simulink model "TCMSSystem"  (R2019b)
settings: configuration reference "ConfigSet_TCMSSystem_Reference" (kept outside this file)
model workspace (MAT data in the model file):
  Prm_TCMSSystem : Simulink.Parameter (value not decoded)
  SampleTime = 0.05
symbols that are objects in the model workspace (value not decoded): Prm_TCMSSystem
undefined symbols (not defined in the file): ADDIntervention, AK1Status, AK2Status, AKContactorStatus, AllDoorsClosed, AllLeftDoorsClosed, AllRightDoorsClosed, APS1Fault, APS1Isolated, APS1OutputVoltage, APS1Status, APS2Fault, APS2Isolated, APS2OutputVoltage, APS2Status, APSKAKContactor, ASCOEnd1, ASCOEnd2, ATBMode, ATCBypassMode, ATCStatusNotOK, ATOMode, ATPLowSpeedCutoutStatus, ATPMode, AuxCompressor, BatteryCurrent, BatteryIsolationContactor, BatteryTemperature, BatteryVoltage, BCG1Fault, BCG1Isolated, BCG1IsolationFailed, BCG1OutputCurrent, BCG1Status, BCG2Fault, BCG2Isolated, BCG2OutputCurrent, BCG2Status, BCGOutputVoltage, BECU1AxleLockedWheelSet1, BECU2AxleLockedWheelSet2, BECUFaulty, BECUMajorFault, BECUMinorFault, BECUStatus, BIC1Inside, BIC1Outside, BIC2Inside, BIC2Outside, Bogie, Bogie1WSPStatus, Bogie2WSPStatus, BogieFaulty, BogieIsolationStatus, BogieSupportedMass, BrakeCylinderPressureGauge, BrakeLoopCBTripped, BrakeLoopOpenTL, BrakeTrainLineStatus, BrakingDemand ... (+215)
libraries: TimersLib x257, simulink x137, LatchesLib x42, VectorOperationsLib x15, TestBenchLib x12, MathOperationsLib x2, FiltersLib x1
(part 14 of 16)

== system TCMSSystem/TCMSSystemPerVehicle/EnabledTCMSVehicle/OutputsPacking/TCMSDisplayOutputs/TCMSMessageEvents/ElectricalSystemFaults/Associated TCMS Fault ID37 ==
  State : Inport
  Bus Creator1 : BusCreator  Inputs=2  OutDataTypeStr=Bus: BD_TCMSSystem_Out_Vehicle_Display_Message  NonVirtualBus=on
  Constant : Constant  Value=MessageID
  Data Type Conversion : DataTypeConversion
  Message : Outport  VectorParamsAs1DForOutWhenUnconnected=off
  wires:
  Data Type Conversion/1 -> Bus Creator1/2  "MessageStatus"
  Constant/1 -> Bus Creator1/1  "MessageID"
  State/1 -> Data Type Conversion/1
  Bus Creator1/1 -> Message/1

== system TCMSSystem/TCMSSystemPerVehicle/EnabledTCMSVehicle/OutputsPacking/TCMSDisplayOutputs/TCMSMessageEvents/ElectricalSystemFaults/Associated TCMS Fault ID38 ==
  State : Inport
  Bus Creator1 : BusCreator  Inputs=2  OutDataTypeStr=Bus: BD_TCMSSystem_Out_Vehicle_Display_Message  NonVirtualBus=on
  Constant : Constant  Value=MessageID
  Data Type Conversion : DataTypeConversion
  Message : Outport  VectorParamsAs1DForOutWhenUnconnected=off
  wires:
  Bus Creator1/1 -> Message/1
  State/1 -> Data Type Conversion/1
  Constant/1 -> Bus Creator1/1  "MessageID"
  Data Type Conversion/1 -> Bus Creator1/2  "MessageStatus"

== system TCMSSystem/TCMSSystemPerVehicle/EnabledTCMSVehicle/OutputsPacking/TCMSDisplayOutputs/TCMSMessageEvents/ElectricalSystemFaults/Associated TCMS Fault ID39 ==
  State : Inport
  Bus Creator1 : BusCreator  Inputs=2  OutDataTypeStr=Bus: BD_TCMSSystem_Out_Vehicle_Display_Message  NonVirtualBus=on
  Constant : Constant  Value=MessageID
  Data Type Conversion : DataTypeConversion
  Message : Outport  VectorParamsAs1DForOutWhenUnconnected=off
  wires:
  Bus Creator1/1 -> Message/1
  State/1 -> Data Type Conversion/1
  Constant/1 -> Bus Creator1/1  "MessageID"
  Data Type Conversion/1 -> Bus Creator1/2  "MessageStatus"

== system TCMSSystem/TCMSSystemPerVehicle/EnabledTCMSVehicle/OutputsPacking/TCMSDisplayOutputs/TCMSMessageEvents/ElectricalSystemFaults/Associated TCMS Fault ID4 ==
  State : Inport
  Bus Creator1 : BusCreator  Inputs=2  OutDataTypeStr=Bus: BD_TCMSSystem_Out_Vehicle_Display_Message  NonVirtualBus=on
  Constant : Constant  Value=MessageID
  Data Type Conversion : DataTypeConversion
  Message : Outport  VectorParamsAs1DForOutWhenUnconnected=off
  wires:
  Data Type Conversion/1 -> Bus Creator1/2  "MessageStatus"
  Constant/1 -> Bus Creator1/1  "MessageID"
  State/1 -> Data Type Conversion/1
  Bus Creator1/1 -> Message/1

== system TCMSSystem/TCMSSystemPerVehicle/EnabledTCMSVehicle/OutputsPacking/TCMSDisplayOutputs/TCMSMessageEvents/ElectricalSystemFaults/Associated TCMS Fault ID40 ==
  State : Inport
  Bus Creator1 : BusCreator  Inputs=2  OutDataTypeStr=Bus: BD_TCMSSystem_Out_Vehicle_Display_Message  NonVirtualBus=on
  Constant : Constant  Value=MessageID
  Data Type Conversion : DataTypeConversion
  Message : Outport  VectorParamsAs1DForOutWhenUnconnected=off
  wires:
  Data Type Conversion/1 -> Bus Creator1/2  "MessageStatus"
  Constant/1 -> Bus Creator1/1  "MessageID"
  State/1 -> Data Type Conversion/1
  Bus Creator1/1 -> Message/1

== system TCMSSystem/TCMSSystemPerVehicle/EnabledTCMSVehicle/OutputsPacking/TCMSDisplayOutputs/TCMSMessageEvents/ElectricalSystemFaults/Associated TCMS Fault ID41 ==
  State : Inport
  Bus Creator1 : BusCreator  Inputs=2  OutDataTypeStr=Bus: BD_TCMSSystem_Out_Vehicle_Display_Message  NonVirtualBus=on
  Constant : Constant  Value=MessageID
  Data Type Conversion : DataTypeConversion
  Message : Outport  VectorParamsAs1DForOutWhenUnconnected=off
  wires:
  Bus Creator1/1 -> Message/1
  State/1 -> Data Type Conversion/1
  Constant/1 -> Bus Creator1/1  "MessageID"
  Data Type Conversion/1 -> Bus Creator1/2  "MessageStatus"

== system TCMSSystem/TCMSSystemPerVehicle/EnabledTCMSVehicle/OutputsPacking/TCMSDisplayOutputs/TCMSMessageEvents/ElectricalSystemFaults/Associated TCMS Fault ID42 ==
  State : Inport
  Bus Creator1 : BusCreator  Inputs=2  OutDataTypeStr=Bus: BD_TCMSSystem_Out_Vehicle_Display_Message  NonVirtualBus=on
  Constant : Constant  Value=MessageID
  Data Type Conversion : DataTypeConversion
  Message : Outport  VectorParamsAs1DForOutWhenUnconnected=off
  wires:
  Data Type Conversion/1 -> Bus Creator1/2  "MessageStatus"
  Constant/1 -> Bus Creator1/1  "MessageID"
  State/1 -> Data Type Conversion/1
  Bus Creator1/1 -> Message/1

== system TCMSSystem/TCMSSystemPerVehicle/EnabledTCMSVehicle/OutputsPacking/TCMSDisplayOutputs/TCMSMessageEvents/ElectricalSystemFaults/Associated TCMS Fault ID5 ==
  State : Inport
  Bus Creator1 : BusCreator  Inputs=2  OutDataTypeStr=Bus: BD_TCMSSystem_Out_Vehicle_Display_Message  NonVirtualBus=on
  Constant : Constant  Value=MessageID
  Data Type Conversion : DataTypeConversion
  Message : Outport  VectorParamsAs1DForOutWhenUnconnected=off
  wires:
  Bus Creator1/1 -> Message/1
  State/1 -> Data Type Conversion/1
  Constant/1 -> Bus Creator1/1  "MessageID"
  Data Type Conversion/1 -> Bus Creator1/2  "MessageStatus"

== system TCMSSystem/TCMSSystemPerVehicle/EnabledTCMSVehicle/OutputsPacking/TCMSDisplayOutputs/TCMSMessageEvents/ElectricalSystemFaults/Associated TCMS Fault ID55 ==
  State : Inport
  Bus Creator1 : BusCreator  Inputs=2  OutDataTypeStr=Bus: BD_TCMSSystem_Out_Vehicle_Display_Message  NonVirtualBus=on
  Constant : Constant  Value=MessageID
  Data Type Conversion : DataTypeConversion
  Message : Outport  VectorParamsAs1DForOutWhenUnconnected=off
  wires:
  Bus Creator1/1 -> Message/1
  State/1 -> Data Type Conversion/1
  Constant/1 -> Bus Creator1/1  "MessageID"
  Data Type Conversion/1 -> Bus Creator1/2  "MessageStatus"

== system TCMSSystem/TCMSSystemPerVehicle/EnabledTCMSVehicle/OutputsPacking/TCMSDisplayOutputs/TCMSMessageEvents/ElectricalSystemFaults/Associated TCMS Fault ID56 ==
  State : Inport
  Bus Creator1 : BusCreator  Inputs=2  OutDataTypeStr=Bus: BD_TCMSSystem_Out_Vehicle_Display_Message  NonVirtualBus=on
  Constant : Constant  Value=MessageID
  Data Type Conversion : DataTypeConversion
  Message : Outport  VectorParamsAs1DForOutWhenUnconnected=off
  wires:
  Data Type Conversion/1 -> Bus Creator1/2  "MessageStatus"
  Constant/1 -> Bus Creator1/1  "MessageID"
  State/1 -> Data Type Conversion/1
  Bus Creator1/1 -> Message/1

== system TCMSSystem/TCMSSystemPerVehicle/EnabledTCMSVehicle/OutputsPacking/TCMSDisplayOutputs/TCMSMessageEvents/ElectricalSystemFaults/Associated TCMS Fault ID58 ==
  State : Inport
  Bus Creator1 : BusCreator  Inputs=2  OutDataTypeStr=Bus: BD_TCMSSystem_Out_Vehicle_Display_Message  NonVirtualBus=on
  Constant : Constant  Value=MessageID
  Data Type Conversion : DataTypeConversion
  Message : Outport  VectorParamsAs1DForOutWhenUnconnected=off
  wires:
  Bus Creator1/1 -> Message/1
  State/1 -> Data Type Conversion/1
  Constant/1 -> Bus Creator1/1  "MessageID"
  Data Type Conversion/1 -> Bus Creator1/2  "MessageStatus"

== system TCMSSystem/TCMSSystemPerVehicle/EnabledTCMSVehicle/OutputsPacking/TCMSDisplayOutputs/TCMSMessageEvents/ElectricalSystemFaults/Associated TCMS Fault ID59 ==
  State : Inport
  Bus Creator1 : BusCreator  Inputs=2  OutDataTypeStr=Bus: BD_TCMSSystem_Out_Vehicle_Display_Message  NonVirtualBus=on
  Constant : Constant  Value=MessageID
  Data Type Conversion : DataTypeConversion
  Message : Outport  VectorParamsAs1DForOutWhenUnconnected=off
  wires:
  Data Type Conversion/1 -> Bus Creator1/2  "MessageStatus"
  Constant/1 -> Bus Creator1/1  "MessageID"
  State/1 -> Data Type Conversion/1
  Bus Creator1/1 -> Message/1

== system TCMSSystem/TCMSSystemPerVehicle/EnabledTCMSVehicle/OutputsPacking/TCMSDisplayOutputs/TCMSMessageEvents/ElectricalSystemFaults/Associated TCMS Fault ID6 ==
  State : Inport
  Bus Creator1 : BusCreator  Inputs=2  OutDataTypeStr=Bus: BD_TCMSSystem_Out_Vehicle_Display_Message  NonVirtualBus=on
  Constant : Constant  Value=MessageID
  Data Type Conversion : DataTypeConversion
  Message : Outport  VectorParamsAs1DForOutWhenUnconnected=off
  wires:
  Data Type Conversion/1 -> Bus Creator1/2  "MessageStatus"
  Constant/1 -> Bus Creator1/1  "MessageID"
  State/1 -> Data Type Conversion/1
  Bus Creator1/1 -> Message/1

== system TCMSSystem/TCMSSystemPerVehicle/EnabledTCMSVehicle/OutputsPacking/TCMSDisplayOutputs/TCMSMessageEvents/ElectricalSystemFaults/Associated TCMS Fault ID60 ==
  State : Inport
  Bus Creator1 : BusCreator  Inputs=2  OutDataTypeStr=Bus: BD_TCMSSystem_Out_Vehicle_Display_Message  NonVirtualBus=on
  Constant : Constant  Value=MessageID
  Data Type Conversion : DataTypeConversion
  Message : Outport  VectorParamsAs1DForOutWhenUnconnected=off
  wires:
  Bus Creator1/1 -> Message/1
  State/1 -> Data Type Conversion/1
  Constant/1 -> Bus Creator1/1  "MessageID"
  Data Type Conversion/1 -> Bus Creator1/2  "MessageStatus"

== system TCMSSystem/TCMSSystemPerVehicle/EnabledTCMSVehicle/OutputsPacking/TCMSDisplayOutputs/TCMSMessageEvents/ElectricalSystemFaults/Associated TCMS Fault ID61 ==
  State : Inport
  Bus Creator1 : BusCreator  Inputs=2  OutDataTypeStr=Bus: BD_TCMSSystem_Out_Vehicle_Display_Message  NonVirtualBus=on
  Constant : Constant  Value=MessageID
  Data Type Conversion : DataTypeConversion
  Message : Outport  VectorParamsAs1DForOutWhenUnconnected=off
  wires:
  Data Type Conversion/1 -> Bus Creator1/2  "MessageStatus"
  Constant/1 -> Bus Creator1/1  "MessageID"
  State/1 -> Data Type Conversion/1
  Bus Creator1/1 -> Message/1

== system TCMSSystem/TCMSSystemPerVehicle/EnabledTCMSVehicle/OutputsPacking/TCMSDisplayOutputs/TCMSMessageEvents/ElectricalSystemFaults/Associated TCMS Fault ID62 ==
  State : Inport
  Bus Creator1 : BusCreator  Inputs=2  OutDataTypeStr=Bus: BD_TCMSSystem_Out_Vehicle_Display_Message  NonVirtualBus=on
  Constant : Constant  Value=MessageID
  Data Type Conversion : DataTypeConversion
  Message : Outport  VectorParamsAs1DForOutWhenUnconnected=off
  wires:
  Data Type Conversion/1 -> Bus Creator1/2  "MessageStatus"
  Constant/1 -> Bus Creator1/1  "MessageID"
  State/1 -> Data Type Conversion/1
  Bus Creator1/1 -> Message/1

== system TCMSSystem/TCMSSystemPerVehicle/EnabledTCMSVehicle/OutputsPacking/TCMSDisplayOutputs/TCMSMessageEvents/ElectricalSystemFaults/Associated TCMS Fault ID63 ==
  State : Inport
  Bus Creator1 : BusCreator  Inputs=2  OutDataTypeStr=Bus: BD_TCMSSystem_Out_Vehicle_Display_Message  NonVirtualBus=on
  Constant : Constant  Value=MessageID
  Data Type Conversion : DataTypeConversion
  Message : Outport  VectorParamsAs1DForOutWhenUnconnected=off
  wires:
  Bus Creator1/1 -> Message/1
  State/1 -> Data Type Conversion/1
  Constant/1 -> Bus Creator1/1  "MessageID"
  Data Type Conversion/1 -> Bus Creator1/2  "MessageStatus"

== system TCMSSystem/TCMSSystemPerVehicle/EnabledTCMSVehicle/OutputsPacking/TCMSDisplayOutputs/TCMSMessageEvents/ElectricalSystemFaults/Associated TCMS Fault ID64 ==
  State : Inport
  Bus Creator1 : BusCreator  Inputs=2  OutDataTypeStr=Bus: BD_TCMSSystem_Out_Vehicle_Display_Message  NonVirtualBus=on
  Constant : Constant  Value=MessageID
  Data Type Conversion : DataTypeConversion
  Message : Outport  VectorParamsAs1DForOutWhenUnconnected=off
  wires:
  Data Type Conversion/1 -> Bus Creator1/2  "MessageStatus"
  Constant/1 -> Bus Creator1/1  "MessageID"
  State/1 -> Data Type Conversion/1
  Bus Creator1/1 -> Message/1

== system TCMSSystem/TCMSSystemPerVehicle/EnabledTCMSVehicle/OutputsPacking/TCMSDisplayOutputs/TCMSMessageEvents/ElectricalSystemFaults/Associated TCMS Fault ID65 ==
  State : Inport
  Bus Creator1 : BusCreator  Inputs=2  OutDataTypeStr=Bus: BD_TCMSSystem_Out_Vehicle_Display_Message  NonVirtualBus=on
  Constant : Constant  Value=MessageID
  Data Type Conversion : DataTypeConversion
  Message : Outport  VectorParamsAs1DForOutWhenUnconnected=off
  wires:
  Bus Creator1/1 -> Message/1
  State/1 -> Data Type Conversion/1
  Constant/1 -> Bus Creator1/1  "MessageID"
  Data Type Conversion/1 -> Bus Creator1/2  "MessageStatus"

== system TCMSSystem/TCMSSystemPerVehicle/EnabledTCMSVehicle/OutputsPacking/TCMSDisplayOutputs/TCMSMessageEvents/ElectricalSystemFaults/Associated TCMS Fault ID66 ==
  State : Inport
  Bus Creator1 : BusCreator  Inputs=2  OutDataTypeStr=Bus: BD_TCMSSystem_Out_Vehicle_Display_Message  NonVirtualBus=on
  Constant : Constant  Value=MessageID
  Data Type Conversion : DataTypeConversion
  Message : Outport  VectorParamsAs1DForOutWhenUnconnected=off
  wires:
  Data Type Conversion/1 -> Bus Creator1/2  "MessageStatus"
  Constant/1 -> Bus Creator1/1  "MessageID"
  State/1 -> Data Type Conversion/1
  Bus Creator1/1 -> Message/1

== system TCMSSystem/TCMSSystemPerVehicle/EnabledTCMSVehicle/OutputsPacking/TCMSDisplayOutputs/TCMSMessageEvents/ElectricalSystemFaults/Associated TCMS Fault ID67 ==
  State : Inport
  Bus Creator1 : BusCreator  Inputs=2  OutDataTypeStr=Bus: BD_TCMSSystem_Out_Vehicle_Display_Message  NonVirtualBus=on
  Constant : Constant  Value=MessageID
  Data Type Conversion : DataTypeConversion
  Message : Outport  VectorParamsAs1DForOutWhenUnconnected=off
  wires:
  Bus Creator1/1 -> Message/1
  State/1 -> Data Type Conversion/1
  Constant/1 -> Bus Creator1/1  "MessageID"
  Data Type Conversion/1 -> Bus Creator1/2  "MessageStatus"

== system TCMSSystem/TCMSSystemPerVehicle/EnabledTCMSVehicle/OutputsPacking/TCMSDisplayOutputs/TCMSMessageEvents/ElectricalSystemFaults/Associated TCMS Fault ID68 ==
  State : Inport
  Bus Creator1 : BusCreator  Inputs=2  OutDataTypeStr=Bus: BD_TCMSSystem_Out_Vehicle_Display_Message  NonVirtualBus=on
  Constant : Constant  Value=MessageID
  Data Type Conversion : DataTypeConversion
  Message : Outport  VectorParamsAs1DForOutWhenUnconnected=off
  wires:
  Data Type Conversion/1 -> Bus Creator1/2  "MessageStatus"
  Constant/1 -> Bus Creator1/1  "MessageID"
  State/1 -> Data Type Conversion/1
  Bus Creator1/1 -> Message/1

== system TCMSSystem/TCMSSystemPerVehicle/EnabledTCMSVehicle/OutputsPacking/TCMSDisplayOutputs/TCMSMessageEvents/ElectricalSystemFaults/Associated TCMS Fault ID69 ==
  State : Inport
  Bus Creator1 : BusCreator  Inputs=2  OutDataTypeStr=Bus: BD_TCMSSystem_Out_Vehicle_Display_Message  NonVirtualBus=on
  Constant : Constant  Value=MessageID
  Data Type Conversion : DataTypeConversion
  Message : Outport  VectorParamsAs1DForOutWhenUnconnected=off
  wires:
  Bus Creator1/1 -> Message/1
  State/1 -> Data Type Conversion/1
  Constant/1 -> Bus Creator1/1  "MessageID"
  Data Type Conversion/1 -> Bus Creator1/2  "MessageStatus"

== system TCMSSystem/TCMSSystemPerVehicle/EnabledTCMSVehicle/OutputsPacking/TCMSDisplayOutputs/TCMSMessageEvents/ElectricalSystemFaults/Associated TCMS Fault ID7 ==
  State : Inport
  Bus Creator1 : BusCreator  Inputs=2  OutDataTypeStr=Bus: BD_TCMSSystem_Out_Vehicle_Display_Message  NonVirtualBus=on
  Constant : Constant  Value=MessageID
  Data Type Conversion : DataTypeConversion
  Message : Outport  VectorParamsAs1DForOutWhenUnconnected=off
  wires:
  Bus Creator1/1 -> Message/1
  State/1 -> Data Type Conversion/1
  Constant/1 -> Bus Creator1/1  "MessageID"
  Data Type Conversion/1 -> Bus Creator1/2  "MessageStatus"

== system TCMSSystem/TCMSSystemPerVehicle/EnabledTCMSVehicle/OutputsPacking/TCMSDisplayOutputs/TCMSMessageEvents/ElectricalSystemFaults/Associated TCMS Fault ID70 ==
  State : Inport
  Bus Creator1 : BusCreator  Inputs=2  OutDataTypeStr=Bus: BD_TCMSSystem_Out_Vehicle_Display_Message  NonVirtualBus=on
  Constant : Constant  Value=MessageID
  Data Type Conversion : DataTypeConversion
  Message : Outport  VectorParamsAs1DForOutWhenUnconnected=off
  wires:
  Data Type Conversion/1 -> Bus Creator1/2  "MessageStatus"
  Constant/1 -> Bus Creator1/1  "MessageID"
  State/1 -> Data Type Conversion/1
  Bus Creator1/1 -> Message/1

== system TCMSSystem/TCMSSystemPerVehicle/EnabledTCMSVehicle/OutputsPacking/TCMSDisplayOutputs/TCMSMessageEvents/ElectricalSystemFaults/Associated TCMS Fault ID71 ==
  State : Inport
  Bus Creator1 : BusCreator  Inputs=2  OutDataTypeStr=Bus: BD_TCMSSystem_Out_Vehicle_Display_Message  NonVirtualBus=on
  Constant : Constant  Value=MessageID
  Data Type Conversion : DataTypeConversion
  Message : Outport  VectorParamsAs1DForOutWhenUnconnected=off
  wires:
  Bus Creator1/1 -> Message/1
  State/1 -> Data Type Conversion/1
  Constant/1 -> Bus Creator1/1  "MessageID"
  Data Type Conversion/1 -> Bus Creator1/2  "MessageStatus"

== system TCMSSystem/TCMSSystemPerVehicle/EnabledTCMSVehicle/OutputsPacking/TCMSDisplayOutputs/TCMSMessageEvents/ElectricalSystemFaults/Associated TCMS Fault ID72 ==
  State : Inport
  Bus Creator1 : BusCreator  Inputs=2  OutDataTypeStr=Bus: BD_TCMSSystem_Out_Vehicle_Display_Message  NonVirtualBus=on
  Constant : Constant  Value=MessageID
  Data Type Conversion : DataTypeConversion
  Message : Outport  VectorParamsAs1DForOutWhenUnconnected=off
  wires:
  Data Type Conversion/1 -> Bus Creator1/2  "MessageStatus"
  Constant/1 -> Bus Creator1/1  "MessageID"
  State/1 -> Data Type Conversion/1
  Bus Creator1/1 -> Message/1

== system TCMSSystem/TCMSSystemPerVehicle/EnabledTCMSVehicle/OutputsPacking/TCMSDisplayOutputs/TCMSMessageEvents/ElectricalSystemFaults/Associated TCMS Fault ID73 ==
  State : Inport
  Bus Creator1 : BusCreator  Inputs=2  OutDataTypeStr=Bus: BD_TCMSSystem_Out_Vehicle_Display_Message  NonVirtualBus=on
  Constant : Constant  Value=MessageID
  Data Type Conversion : DataTypeConversion
  Message : Outport  VectorParamsAs1DForOutWhenUnconnected=off
  wires:
  Bus Creator1/1 -> Message/1
  State/1 -> Data Type Conversion/1
  Constant/1 -> Bus Creator1/1  "MessageID"
  Data Type Conversion/1 -> Bus Creator1/2  "MessageStatus"

== system TCMSSystem/TCMSSystemPerVehicle/EnabledTCMSVehicle/OutputsPacking/TCMSDisplayOutputs/TCMSMessageEvents/ElectricalSystemFaults/Associated TCMS Fault ID74 ==
  State : Inport
  Bus Creator1 : BusCreator  Inputs=2  OutDataTypeStr=Bus: BD_TCMSSystem_Out_Vehicle_Display_Message  NonVirtualBus=on
  Constant : Constant  Value=MessageID
  Data Type Conversion : DataTypeConversion
  Message : Outport  VectorParamsAs1DForOutWhenUnconnected=off
  wires:
  Bus Creator1/1 -> Message/1
  State/1 -> Data Type Conversion/1
  Constant/1 -> Bus Creator1/1  "MessageID"
  Data Type Conversion/1 -> Bus Creator1/2  "MessageStatus"

== system TCMSSystem/TCMSSystemPerVehicle/EnabledTCMSVehicle/OutputsPacking/TCMSDisplayOutputs/TCMSMessageEvents/ElectricalSystemFaults/Associated TCMS Fault ID75 ==
  State : Inport
  Bus Creator1 : BusCreator  Inputs=2  OutDataTypeStr=Bus: BD_TCMSSystem_Out_Vehicle_Display_Message  NonVirtualBus=on
  Constant : Constant  Value=MessageID
  Data Type Conversion : DataTypeConversion
  Message : Outport  VectorParamsAs1DForOutWhenUnconnected=off
  wires:
  Data Type Conversion/1 -> Bus Creator1/2  "MessageStatus"
  Constant/1 -> Bus Creator1/1  "MessageID"
  State/1 -> Data Type Conversion/1
  Bus Creator1/1 -> Message/1

== system TCMSSystem/TCMSSystemPerVehicle/EnabledTCMSVehicle/OutputsPacking/TCMSDisplayOutputs/TCMSMessageEvents/ElectricalSystemFaults/Associated TCMS Fault ID76 ==
  State : Inport
  Bus Creator1 : BusCreator  Inputs=2  OutDataTypeStr=Bus: BD_TCMSSystem_Out_Vehicle_Display_Message  NonVirtualBus=on
  Constant : Constant  Value=MessageID
  Data Type Conversion : DataTypeConversion
  Message : Outport  VectorParamsAs1DForOutWhenUnconnected=off
  wires:
  Bus Creator1/1 -> Message/1
  State/1 -> Data Type Conversion/1
  Constant/1 -> Bus Creator1/1  "MessageID"
  Data Type Conversion/1 -> Bus Creator1/2  "MessageStatus"

== system TCMSSystem/TCMSSystemPerVehicle/EnabledTCMSVehicle/OutputsPacking/TCMSDisplayOutputs/TCMSMessageEvents/ElectricalSystemFaults/Associated TCMS Fault ID77 ==
  State : Inport
  Bus Creator1 : BusCreator  Inputs=2  OutDataTypeStr=Bus: BD_TCMSSystem_Out_Vehicle_Display_Message  NonVirtualBus=on
  Constant : Constant  Value=MessageID
  Data Type Conversion : DataTypeConversion
  Message : Outport  VectorParamsAs1DForOutWhenUnconnected=off
  wires:
  Data Type Conversion/1 -> Bus Creator1/2  "MessageStatus"
  Constant/1 -> Bus Creator1/1  "MessageID"
  State/1 -> Data Type Conversion/1
  Bus Creator1/1 -> Message/1

== system TCMSSystem/TCMSSystemPerVehicle/EnabledTCMSVehicle/OutputsPacking/TCMSDisplayOutputs/TCMSMessageEvents/ElectricalSystemFaults/Associated TCMS Fault ID78 ==
  State : Inport
  Bus Creator1 : BusCreator  Inputs=2  OutDataTypeStr=Bus: BD_TCMSSystem_Out_Vehicle_Display_Message  NonVirtualBus=on
  Constant : Constant  Value=MessageID
  Data Type Conversion : DataTypeConversion
  Message : Outport  VectorParamsAs1DForOutWhenUnconnected=off
  wires:
  Bus Creator1/1 -> Message/1
  State/1 -> Data Type Conversion/1
  Constant/1 -> Bus Creator1/1  "MessageID"
  Data Type Conversion/1 -> Bus Creator1/2  "MessageStatus"

== system TCMSSystem/TCMSSystemPerVehicle/EnabledTCMSVehicle/OutputsPacking/TCMSDisplayOutputs/TCMSMessageEvents/ElectricalSystemFaults/Associated TCMS Fault ID79 ==
  State : Inport
  Bus Creator1 : BusCreator  Inputs=2  OutDataTypeStr=Bus: BD_TCMSSystem_Out_Vehicle_Display_Message  NonVirtualBus=on
  Constant : Constant  Value=MessageID
  Data Type Conversion : DataTypeConversion
  Message : Outport  VectorParamsAs1DForOutWhenUnconnected=off
  wires:
  Data Type Conversion/1 -> Bus Creator1/2  "MessageStatus"
  Constant/1 -> Bus Creator1/1  "MessageID"
  State/1 -> Data Type Conversion/1
  Bus Creator1/1 -> Message/1

== system TCMSSystem/TCMSSystemPerVehicle/EnabledTCMSVehicle/OutputsPacking/TCMSDisplayOutputs/TCMSMessageEvents/ElectricalSystemFaults/Associated TCMS Fault ID8 ==
  State : Inport
  Bus Creator1 : BusCreator  Inputs=2  OutDataTypeStr=Bus: BD_TCMSSystem_Out_Vehicle_Display_Message  NonVirtualBus=on
  Constant : Constant  Value=MessageID
  Data Type Conversion : DataTypeConversion
  Message : Outport  VectorParamsAs1DForOutWhenUnconnected=off
  wires:
  Data Type Conversion/1 -> Bus Creator1/2  "MessageStatus"
  Constant/1 -> Bus Creator1/1  "MessageID"
  State/1 -> Data Type Conversion/1
  Bus Creator1/1 -> Message/1

== system TCMSSystem/TCMSSystemPerVehicle/EnabledTCMSVehicle/OutputsPacking/TCMSDisplayOutputs/TCMSMessageEvents/ElectricalSystemFaults/Associated TCMS Fault ID89 ==
  State : Inport
  Bus Creator1 : BusCreator  Inputs=2  OutDataTypeStr=Bus: BD_TCMSSystem_Out_Vehicle_Display_Message  NonVirtualBus=on
  Constant : Constant  Value=MessageID
  Data Type Conversion : DataTypeConversion
  Message : Outport  VectorParamsAs1DForOutWhenUnconnected=off
  wires:
  Bus Creator1/1 -> Message/1
  State/1 -> Data Type Conversion/1
  Constant/1 -> Bus Creator1/1  "MessageID"
  Data Type Conversion/1 -> Bus Creator1/2  "MessageStatus"

== system TCMSSystem/TCMSSystemPerVehicle/EnabledTCMSVehicle/OutputsPacking/TCMSDisplayOutputs/TCMSMessageEvents/ElectricalSystemFaults/Associated TCMS Fault ID9 ==
  State : Inport
  Bus Creator1 : BusCreator  Inputs=2  OutDataTypeStr=Bus: BD_TCMSSystem_Out_Vehicle_Display_Message  NonVirtualBus=on
  Constant : Constant  Value=MessageID
  Data Type Conversion : DataTypeConversion
  Message : Outport  VectorParamsAs1DForOutWhenUnconnected=off
  wires:
  Bus Creator1/1 -> Message/1
  State/1 -> Data Type Conversion/1
  Constant/1 -> Bus Creator1/1  "MessageID"
  Data Type Conversion/1 -> Bus Creator1/2  "MessageStatus"

== system TCMSSystem/TCMSSystemPerVehicle/EnabledTCMSVehicle/OutputsPacking/TCMSDisplayOutputs/TCMSMessageEvents/ElectricalSystemFaults/Associated TCMS Fault ID90 ==
  State : Inport
  Bus Creator1 : BusCreator  Inputs=2  OutDataTypeStr=Bus: BD_TCMSSystem_Out_Vehicle_Display_Message  NonVirtualBus=on
  Constant : Constant  Value=MessageID
  Data Type Conversion : DataTypeConversion
  Message : Outport  VectorParamsAs1DForOutWhenUnconnected=off
  wires:
  Bus Creator1/1 -> Message/1
  State/1 -> Data Type Conversion/1
  Constant/1 -> Bus Creator1/1  "MessageID"
  Data Type Conversion/1 -> Bus Creator1/2  "MessageStatus"

== system TCMSSystem/TCMSSystemPerVehicle/EnabledTCMSVehicle/OutputsPacking/TCMSDisplayOutputs/TCMSMessageEvents/ElectricalSystemFaults/Associated TCMS Fault ID91 ==
  State : Inport
  Bus Creator1 : BusCreator  Inputs=2  OutDataTypeStr=Bus: BD_TCMSSystem_Out_Vehicle_Display_Message  NonVirtualBus=on
  Constant : Constant  Value=MessageID
  Data Type Conversion : DataTypeConversion
  Message : Outport  VectorParamsAs1DForOutWhenUnconnected=off
  wires:
  Data Type Conversion/1 -> Bus Creator1/2  "MessageStatus"
  Constant/1 -> Bus Creator1/1  "MessageID"
  State/1 -> Data Type Conversion/1
  Bus Creator1/1 -> Message/1

== system TCMSSystem/TCMSSystemPerVehicle/EnabledTCMSVehicle/OutputsPacking/TCMSDisplayOutputs/TCMSMessageEvents/ElectricalSystemFaults/Associated TCMS Fault ID92 ==
  State : Inport
  Bus Creator1 : BusCreator  Inputs=2  OutDataTypeStr=Bus: BD_TCMSSystem_Out_Vehicle_Display_Message  NonVirtualBus=on
  Constant : Constant  Value=MessageID
  Data Type Conversion : DataTypeConversion
  Message : Outport  VectorParamsAs1DForOutWhenUnconnected=off
  wires:
  Data Type Conversion/1 -> Bus Creator1/2  "MessageStatus"
  Constant/1 -> Bus Creator1/1  "MessageID"
  State/1 -> Data Type Conversion/1
  Bus Creator1/1 -> Message/1

== system TCMSSystem/TCMSSystemPerVehicle/EnabledTCMSVehicle/OutputsPacking/TCMSDisplayOutputs/TCMSMessageEvents/ElectricalSystemFaults/Associated TCMS Fault ID93 ==
  State : Inport
  Bus Creator1 : BusCreator  Inputs=2  OutDataTypeStr=Bus: BD_TCMSSystem_Out_Vehicle_Display_Message  NonVirtualBus=on
  Constant : Constant  Value=MessageID
  Data Type Conversion : DataTypeConversion
  Message : Outport  VectorParamsAs1DForOutWhenUnconnected=off
  wires:
  Bus Creator1/1 -> Message/1
  State/1 -> Data Type Conversion/1
  Constant/1 -> Bus Creator1/1  "MessageID"
  Data Type Conversion/1 -> Bus Creator1/2  "MessageStatus"

== system TCMSSystem/TCMSSystemPerVehicle/EnabledTCMSVehicle/OutputsPacking/TCMSDisplayOutputs/TCMSMessageEvents/ElectricalSystemFaults/Associated TCMS Fault ID94 ==
  State : Inport
  Bus Creator1 : BusCreator  Inputs=2  OutDataTypeStr=Bus: BD_TCMSSystem_Out_Vehicle_Display_Message  NonVirtualBus=on
  Constant : Constant  Value=MessageID
  Data Type Conversion : DataTypeConversion
  Message : Outport  VectorParamsAs1DForOutWhenUnconnected=off
  wires:
  Data Type Conversion/1 -> Bus Creator1/2  "MessageStatus"
  Constant/1 -> Bus Creator1/1  "MessageID"
  State/1 -> Data Type Conversion/1
  Bus Creator1/1 -> Message/1

== system TCMSSystem/TCMSSystemPerVehicle/EnabledTCMSVehicle/OutputsPacking/TCMSDisplayOutputs/TCMSMessageEvents/ElectricalSystemFaults/Associated TCMS Fault ID95 ==
  State : Inport
  Bus Creator1 : BusCreator  Inputs=2  OutDataTypeStr=Bus: BD_TCMSSystem_Out_Vehicle_Display_Message  NonVirtualBus=on
  Constant : Constant  Value=MessageID
  Data Type Conversion : DataTypeConversion
  Message : Outport  VectorParamsAs1DForOutWhenUnconnected=off
  wires:
  Data Type Conversion/1 -> Bus Creator1/2  "MessageStatus"
  Constant/1 -> Bus Creator1/1  "MessageID"
  State/1 -> Data Type Conversion/1
  Bus Creator1/1 -> Message/1

== system TCMSSystem/TCMSSystemPerVehicle/EnabledTCMSVehicle/OutputsPacking/TCMSDisplayOutputs/TCMSMessageEvents/ElectricalSystemFaults/Associated TCMS Fault ID96 ==
  State : Inport
  Bus Creator1 : BusCreator  Inputs=2  OutDataTypeStr=Bus: BD_TCMSSystem_Out_Vehicle_Display_Message  NonVirtualBus=on
  Constant : Constant  Value=MessageID
  Data Type Conversion : DataTypeConversion
  Message : Outport  VectorParamsAs1DForOutWhenUnconnected=off
  wires:
  Bus Creator1/1 -> Message/1
  State/1 -> Data Type Conversion/1
  Constant/1 -> Bus Creator1/1  "MessageID"
  Data Type Conversion/1 -> Bus Creator1/2  "MessageStatus"

== system TCMSSystem/TCMSSystemPerVehicle/EnabledTCMSVehicle/OutputsPacking/TCMSDisplayOutputs/TCMSMessageEvents/MessageShortList/Associated TCMS Fault ID ==
  State : Inport
  Bus Creator1 : BusCreator  Inputs=2  OutDataTypeStr=Bus: BD_TCMS_Out_Vehicle_Message  NonVirtualBus=on
  Constant : Constant  Value=MessageID
  Data Type Conversion : DataTypeConversion
  Message : Outport  VectorParamsAs1DForOutWhenUnconnected=off
  wires:
  Data Type Conversion/1 -> Bus Creator1/2  "MessageStatus"
  Constant/1 -> Bus Creator1/1  "MessageID"
  State/1 -> Data Type Conversion/1
  Bus Creator1/1 -> Message/1

== system TCMSSystem/TCMSSystemPerVehicle/EnabledTCMSVehicle/OutputsPacking/TCMSDisplayOutputs/TCMSMessageEvents/MessageShortList/For Each Subsystem ==
  Message : Inport  Partition=on  PartitionDimension=1  PartitionWidth=1  PartitionOffset=0
  Bus Selector : BusSelector  OutputSignals=MessageStatus
  For Each : ForEach  DisableCoverage=on
  MessageStatus : Outport  ConcatenationDimension=1
  wires:
  Message/1 -> Bus Selector/1
  Bus Selector/1 -> MessageStatus/1  "<MessageStatus>"

== system TCMSSystem/TCMSSystemPerVehicle/EnabledTCMSVehicle/OutputsPacking/TCMSDisplayOutputs/TCMSMessageEvents/MessageShortList/TCMS Message Index List ==
  note: ensures that events that were
      | previously in the list, don't move
      | around in the order
  note: finds non zero elements pads out to 10 elements
      | 10 is hard coded currently
  Status : Inport
  Delay : Delay  DelayLength=1  InitialCondition=zeros(1,10)
  pad : MATLAB Function  TreatAsAtomicUnit=on
  pad1 : MATLAB Function  TreatAsAtomicUnit=on
  IndexList : Outport  VectorParamsAs1DForOutWhenUnconnected=off
  wires:
  pad/1(y) -> pad1/1(u)
  Delay/1 -> pad1/2(y_prev)
  Status/1 -> pad/1(u)  "status"
  pad1/1(y) -> Delay/1, IndexList/1

== system TCMSSystem/TCMSSystemPerVehicle/EnabledTCMSVehicle/OutputsPacking/TCMSDisplayOutputs/TCMSMessageEvents/MiscellaneousFaults/Associated TCMS Fault ID1 ==
  State : Inport
  Bus Creator1 : BusCreator  Inputs=2  OutDataTypeStr=Bus: BD_TCMSSystem_Out_Vehicle_Display_Message  NonVirtualBus=on
  Constant : Constant  Value=MessageID
  Data Type Conversion : DataTypeConversion
  Message : Outport  VectorParamsAs1DForOutWhenUnconnected=off
  wires:
  Data Type Conversion/1 -> Bus Creator1/2  "MessageStatus"
  Constant/1 -> Bus Creator1/1  "MessageID"
  State/1 -> Data Type Conversion/1
  Bus Creator1/1 -> Message/1

== system TCMSSystem/TCMSSystemPerVehicle/EnabledTCMSVehicle/OutputsPacking/TCMSDisplayOutputs/TCMSMessageEvents/MiscellaneousFaults/Associated TCMS Fault ID102 ==
  State : Inport
  Bus Creator1 : BusCreator  Inputs=2  OutDataTypeStr=Bus: BD_TCMSSystem_Out_Vehicle_Display_Message  NonVirtualBus=on
  Constant : Constant  Value=MessageID
  Data Type Conversion : DataTypeConversion
  Message : Outport  VectorParamsAs1DForOutWhenUnconnected=off
  wires:
  Bus Creator1/1 -> Message/1
  State/1 -> Data Type Conversion/1
  Constant/1 -> Bus Creator1/1  "MessageID"
  Data Type Conversion/1 -> Bus Creator1/2  "MessageStatus"

== system TCMSSystem/TCMSSystemPerVehicle/EnabledTCMSVehicle/OutputsPacking/TCMSDisplayOutputs/TCMSMessageEvents/MiscellaneousFaults/Associated TCMS Fault ID103 ==
  State : Inport
  Bus Creator1 : BusCreator  Inputs=2  OutDataTypeStr=Bus: BD_TCMSSystem_Out_Vehicle_Display_Message  NonVirtualBus=on
  Constant : Constant  Value=MessageID
  Data Type Conversion : DataTypeConversion
  Message : Outport  VectorParamsAs1DForOutWhenUnconnected=off
  wires:
  Data Type Conversion/1 -> Bus Creator1/2  "MessageStatus"
  Constant/1 -> Bus Creator1/1  "MessageID"
  State/1 -> Data Type Conversion/1
  Bus Creator1/1 -> Message/1

== system TCMSSystem/TCMSSystemPerVehicle/EnabledTCMSVehicle/OutputsPacking/TCMSDisplayOutputs/TCMSMessageEvents/MiscellaneousFaults/Associated TCMS Fault ID104 ==
  State : Inport
  Bus Creator1 : BusCreator  Inputs=2  OutDataTypeStr=Bus: BD_TCMSSystem_Out_Vehicle_Display_Message  NonVirtualBus=on
  Constant : Constant  Value=MessageID
  Data Type Conversion : DataTypeConversion
  Message : Outport  VectorParamsAs1DForOutWhenUnconnected=off
  wires:
  Bus Creator1/1 -> Message/1
  State/1 -> Data Type Conversion/1
  Constant/1 -> Bus Creator1/1  "MessageID"
  Data Type Conversion/1 -> Bus Creator1/2  "MessageStatus"

== system TCMSSystem/TCMSSystemPerVehicle/EnabledTCMSVehicle/OutputsPacking/TCMSDisplayOutputs/TCMSMessageEvents/MiscellaneousFaults/Associated TCMS Fault ID105 ==
  State : Inport
  Bus Creator1 : BusCreator  Inputs=2  OutDataTypeStr=Bus: BD_TCMSSystem_Out_Vehicle_Display_Message  NonVirtualBus=on
  Constant : Constant  Value=MessageID
  Data Type Conversion : DataTypeConversion
  Message : Outport  VectorParamsAs1DForOutWhenUnconnected=off
  wires:
  Data Type Conversion/1 -> Bus Creator1/2  "MessageStatus"
  Constant/1 -> Bus Creator1/1  "MessageID"
  State/1 -> Data Type Conversion/1
  Bus Creator1/1 -> Message/1

== system TCMSSystem/TCMSSystemPerVehicle/EnabledTCMSVehicle/OutputsPacking/TCMSDisplayOutputs/TCMSMessageEvents/MiscellaneousFaults/Associated TCMS Fault ID106 ==
  State : Inport
  Bus Creator1 : BusCreator  Inputs=2  OutDataTypeStr=Bus: BD_TCMSSystem_Out_Vehicle_Display_Message  NonVirtualBus=on
  Constant : Constant  Value=MessageID
  Data Type Conversion : DataTypeConversion
  Message : Outport  VectorParamsAs1DForOutWhenUnconnected=off
  wires:
  Bus Creator1/1 -> Message/1
  State/1 -> Data Type Conversion/1
  Constant/1 -> Bus Creator1/1  "MessageID"
  Data Type Conversion/1 -> Bus Creator1/2  "MessageStatus"

== system TCMSSystem/TCMSSystemPerVehicle/EnabledTCMSVehicle/OutputsPacking/TCMSDisplayOutputs/TCMSMessageEvents/MiscellaneousFaults/Associated TCMS Fault ID107 ==
  State : Inport
  Bus Creator1 : BusCreator  Inputs=2  OutDataTypeStr=Bus: BD_TCMSSystem_Out_Vehicle_Display_Message  NonVirtualBus=on
  Constant : Constant  Value=MessageID
  Data Type Conversion : DataTypeConversion
  Message : Outport  VectorParamsAs1DForOutWhenUnconnected=off
  wires:
  Data Type Conversion/1 -> Bus Creator1/2  "MessageStatus"
  Constant/1 -> Bus Creator1/1  "MessageID"
  State/1 -> Data Type Conversion/1
  Bus Creator1/1 -> Message/1

== system TCMSSystem/TCMSSystemPerVehicle/EnabledTCMSVehicle/OutputsPacking/TCMSDisplayOutputs/TCMSMessageEvents/MiscellaneousFaults/Associated TCMS Fault ID108 ==
  State : Inport
  Bus Creator1 : BusCreator  Inputs=2  OutDataTypeStr=Bus: BD_TCMSSystem_Out_Vehicle_Display_Message  NonVirtualBus=on
  Constant : Constant  Value=MessageID
  Data Type Conversion : DataTypeConversion
  Message : Outport  VectorParamsAs1DForOutWhenUnconnected=off
  wires:
  Bus Creator1/1 -> Message/1
  State/1 -> Data Type Conversion/1
  Constant/1 -> Bus Creator1/1  "MessageID"
  Data Type Conversion/1 -> Bus Creator1/2  "MessageStatus"

== system TCMSSystem/TCMSSystemPerVehicle/EnabledTCMSVehicle/OutputsPacking/TCMSDisplayOutputs/TCMSMessageEvents/New46EventsMessage/Associated TCMS Fault ID1 ==
  State : Inport
  Bus Creator1 : BusCreator  Inputs=2  OutDataTypeStr=Bus: BD_TCMSSystem_Out_Vehicle_Display_Message  NonVirtualBus=on
  Constant : Constant  Value=MessageID
  Data Type Conversion : DataTypeConversion
  Message : Outport  VectorParamsAs1DForOutWhenUnconnected=off
  wires:
  Bus Creator1/1 -> Message/1
  State/1 -> Data Type Conversion/1
  Constant/1 -> Bus Creator1/1  "MessageID"
  Data Type Conversion/1 -> Bus Creator1/2  "MessageStatus"

== system TCMSSystem/TCMSSystemPerVehicle/EnabledTCMSVehicle/OutputsPacking/TCMSDisplayOutputs/TCMSMessageEvents/New46EventsMessage/Associated TCMS Fault ID11 ==
  State : Inport
  Bus Creator1 : BusCreator  Inputs=2  OutDataTypeStr=Bus: BD_TCMSSystem_Out_Vehicle_Display_Message  NonVirtualBus=on
  Constant : Constant  Value=MessageID
  Data Type Conversion : DataTypeConversion
  Message : Outport  VectorParamsAs1DForOutWhenUnconnected=off
  wires:
  Bus Creator1/1 -> Message/1
  State/1 -> Data Type Conversion/1
  Constant/1 -> Bus Creator1/1  "MessageID"
  Data Type Conversion/1 -> Bus Creator1/2  "MessageStatus"

== system TCMSSystem/TCMSSystemPerVehicle/EnabledTCMSVehicle/OutputsPacking/TCMSDisplayOutputs/TCMSMessageEvents/New46EventsMessage/Associated TCMS Fault ID12 ==
  State : Inport
  Bus Creator1 : BusCreator  Inputs=2  OutDataTypeStr=Bus: BD_TCMSSystem_Out_Vehicle_Display_Message  NonVirtualBus=on
  Constant : Constant  Value=MessageID
  Data Type Conversion : DataTypeConversion
  Message : Outport  VectorParamsAs1DForOutWhenUnconnected=off
  wires:
  Bus Creator1/1 -> Message/1
  State/1 -> Data Type Conversion/1
  Constant/1 -> Bus Creator1/1  "MessageID"
  Data Type Conversion/1 -> Bus Creator1/2  "MessageStatus"

== system TCMSSystem/TCMSSystemPerVehicle/EnabledTCMSVehicle/OutputsPacking/TCMSDisplayOutputs/TCMSMessageEvents/New46EventsMessage/Associated TCMS Fault ID16 ==
  State : Inport
  Bus Creator1 : BusCreator  Inputs=2  OutDataTypeStr=Bus: BD_TCMSSystem_Out_Vehicle_Display_Message  NonVirtualBus=on
  Constant : Constant  Value=MessageID
  Data Type Conversion : DataTypeConversion
  Message : Outport  VectorParamsAs1DForOutWhenUnconnected=off
  wires:
  Bus Creator1/1 -> Message/1
  State/1 -> Data Type Conversion/1
  Constant/1 -> Bus Creator1/1  "MessageID"
  Data Type Conversion/1 -> Bus Creator1/2  "MessageStatus"

== system TCMSSystem/TCMSSystemPerVehicle/EnabledTCMSVehicle/OutputsPacking/TCMSDisplayOutputs/TCMSMessageEvents/New46EventsMessage/Associated TCMS Fault ID17 ==
  State : Inport
  Bus Creator1 : BusCreator  Inputs=2  OutDataTypeStr=Bus: BD_TCMSSystem_Out_Vehicle_Display_Message  NonVirtualBus=on
  Constant : Constant  Value=MessageID
  Data Type Conversion : DataTypeConversion
  Message : Outport  VectorParamsAs1DForOutWhenUnconnected=off
  wires:
  Data Type Conversion/1 -> Bus Creator1/2  "MessageStatus"
  Constant/1 -> Bus Creator1/1  "MessageID"
  State/1 -> Data Type Conversion/1
  Bus Creator1/1 -> Message/1

== system TCMSSystem/TCMSSystemPerVehicle/EnabledTCMSVehicle/OutputsPacking/TCMSDisplayOutputs/TCMSMessageEvents/New46EventsMessage/Associated TCMS Fault ID18 ==
  State : Inport
  Bus Creator1 : BusCreator  Inputs=2  OutDataTypeStr=Bus: BD_TCMSSystem_Out_Vehicle_Display_Message  NonVirtualBus=on
  Constant : Constant  Value=MessageID
  Data Type Conversion : DataTypeConversion
  Message : Outport  VectorParamsAs1DForOutWhenUnconnected=off
  wires:
  Data Type Conversion/1 -> Bus Creator1/2  "MessageStatus"
  Constant/1 -> Bus Creator1/1  "MessageID"
  State/1 -> Data Type Conversion/1
  Bus Creator1/1 -> Message/1

== system TCMSSystem/TCMSSystemPerVehicle/EnabledTCMSVehicle/OutputsPacking/TCMSDisplayOutputs/TCMSMessageEvents/New46EventsMessage/Associated TCMS Fault ID19 ==
  State : Inport
  Bus Creator1 : BusCreator  Inputs=2  OutDataTypeStr=Bus: BD_TCMSSystem_Out_Vehicle_Display_Message  NonVirtualBus=on
  Constant : Constant  Value=MessageID
  Data Type Conversion : DataTypeConversion
  Message : Outport  VectorParamsAs1DForOutWhenUnconnected=off
  wires:
  Bus Creator1/1 -> Message/1
  State/1 -> Data Type Conversion/1
  Constant/1 -> Bus Creator1/1  "MessageID"
  Data Type Conversion/1 -> Bus Creator1/2  "MessageStatus"

== system TCMSSystem/TCMSSystemPerVehicle/EnabledTCMSVehicle/OutputsPacking/TCMSDisplayOutputs/TCMSMessageEvents/New46EventsMessage/Associated TCMS Fault ID2 ==
  State : Inport
  Bus Creator1 : BusCreator  Inputs=2  OutDataTypeStr=Bus: BD_TCMSSystem_Out_Vehicle_Display_Message  NonVirtualBus=on
  Constant : Constant  Value=MessageID
  Data Type Conversion : DataTypeConversion
  Message : Outport  VectorParamsAs1DForOutWhenUnconnected=off
  wires:
  Data Type Conversion/1 -> Bus Creator1/2  "MessageStatus"
  Constant/1 -> Bus Creator1/1  "MessageID"
  State/1 -> Data Type Conversion/1
  Bus Creator1/1 -> Message/1

== system TCMSSystem/TCMSSystemPerVehicle/EnabledTCMSVehicle/OutputsPacking/TCMSDisplayOutputs/TCMSMessageEvents/New46EventsMessage/Associated TCMS Fault ID20 ==
  State : Inport
  Bus Creator1 : BusCreator  Inputs=2  OutDataTypeStr=Bus: BD_TCMSSystem_Out_Vehicle_Display_Message  NonVirtualBus=on
  Constant : Constant  Value=MessageID
  Data Type Conversion : DataTypeConversion
  Message : Outport  VectorParamsAs1DForOutWhenUnconnected=off
  wires:
  Data Type Conversion/1 -> Bus Creator1/2  "MessageStatus"
  Constant/1 -> Bus Creator1/1  "MessageID"
  State/1 -> Data Type Conversion/1
  Bus Creator1/1 -> Message/1

== system TCMSSystem/TCMSSystemPerVehicle/EnabledTCMSVehicle/OutputsPacking/TCMSDisplayOutputs/TCMSMessageEvents/New46EventsMessage/Associated TCMS Fault ID21 ==
  State : Inport
  Bus Creator1 : BusCreator  Inputs=2  OutDataTypeStr=Bus: BD_TCMSSystem_Out_Vehicle_Display_Message  NonVirtualBus=on
  Constant : Constant  Value=MessageID
  Data Type Conversion : DataTypeConversion
  Message : Outport  VectorParamsAs1DForOutWhenUnconnected=off
  wires:
  Bus Creator1/1 -> Message/1
  State/1 -> Data Type Conversion/1
  Constant/1 -> Bus Creator1/1  "MessageID"
  Data Type Conversion/1 -> Bus Creator1/2  "MessageStatus"

== system TCMSSystem/TCMSSystemPerVehicle/EnabledTCMSVehicle/OutputsPacking/TCMSDisplayOutputs/TCMSMessageEvents/New46EventsMessage/Associated TCMS Fault ID23 ==
  State : Inport
  Bus Creator1 : BusCreator  Inputs=2  OutDataTypeStr=Bus: BD_TCMSSystem_Out_Vehicle_Display_Message  NonVirtualBus=on
  Constant : Constant  Value=MessageID
  Data Type Conversion : DataTypeConversion
  Message : Outport  VectorParamsAs1DForOutWhenUnconnected=off
  wires:
  Bus Creator1/1 -> Message/1
  State/1 -> Data Type Conversion/1
  Constant/1 -> Bus Creator1/1  "MessageID"
  Data Type Conversion/1 -> Bus Creator1/2  "MessageStatus"

== system TCMSSystem/TCMSSystemPerVehicle/EnabledTCMSVehicle/OutputsPacking/TCMSDisplayOutputs/TCMSMessageEvents/New46EventsMessage/Associated TCMS Fault ID24 ==
  State : Inport
  Bus Creator1 : BusCreator  Inputs=2  OutDataTypeStr=Bus: BD_TCMSSystem_Out_Vehicle_Display_Message  NonVirtualBus=on
  Constant : Constant  Value=MessageID
  Data Type Conversion : DataTypeConversion
  Message : Outport  VectorParamsAs1DForOutWhenUnconnected=off
  wires:
  Data Type Conversion/1 -> Bus Creator1/2  "MessageStatus"
  Constant/1 -> Bus Creator1/1  "MessageID"
  State/1 -> Data Type Conversion/1
  Bus Creator1/1 -> Message/1

== system TCMSSystem/TCMSSystemPerVehicle/EnabledTCMSVehicle/OutputsPacking/TCMSDisplayOutputs/TCMSMessageEvents/New46EventsMessage/Associated TCMS Fault ID25 ==
  State : Inport
  Bus Creator1 : BusCreator  Inputs=2  OutDataTypeStr=Bus: BD_TCMSSystem_Out_Vehicle_Display_Message  NonVirtualBus=on
  Constant : Constant  Value=MessageID
  Data Type Conversion : DataTypeConversion
  Message : Outport  VectorParamsAs1DForOutWhenUnconnected=off
  wires:
  Bus Creator1/1 -> Message/1
  State/1 -> Data Type Conversion/1
  Constant/1 -> Bus Creator1/1  "MessageID"
  Data Type Conversion/1 -> Bus Creator1/2  "MessageStatus"

== system TCMSSystem/TCMSSystemPerVehicle/EnabledTCMSVehicle/OutputsPacking/TCMSDisplayOutputs/TCMSMessageEvents/New46EventsMessage/Associated TCMS Fault ID26 ==
  State : Inport
  Bus Creator1 : BusCreator  Inputs=2  OutDataTypeStr=Bus: BD_TCMSSystem_Out_Vehicle_Display_Message  NonVirtualBus=on
  Constant : Constant  Value=MessageID
  Data Type Conversion : DataTypeConversion
  Message : Outport  VectorParamsAs1DForOutWhenUnconnected=off
  wires:
  Data Type Conversion/1 -> Bus Creator1/2  "MessageStatus"
  Constant/1 -> Bus Creator1/1  "MessageID"
  State/1 -> Data Type Conversion/1
  Bus Creator1/1 -> Message/1

== system TCMSSystem/TCMSSystemPerVehicle/EnabledTCMSVehicle/OutputsPacking/TCMSDisplayOutputs/TCMSMessageEvents/New46EventsMessage/Associated TCMS Fault ID27 ==
  State : Inport
  Bus Creator1 : BusCreator  Inputs=2  OutDataTypeStr=Bus: BD_TCMSSystem_Out_Vehicle_Display_Message  NonVirtualBus=on
  Constant : Constant  Value=MessageID
  Data Type Conversion : DataTypeConversion
  Message : Outport  VectorParamsAs1DForOutWhenUnconnected=off
  wires:
  Data Type Conversion/1 -> Bus Creator1/2  "MessageStatus"
  Constant/1 -> Bus Creator1/1  "MessageID"
  State/1 -> Data Type Conversion/1
  Bus Creator1/1 -> Message/1

== system TCMSSystem/TCMSSystemPerVehicle/EnabledTCMSVehicle/OutputsPacking/TCMSDisplayOutputs/TCMSMessageEvents/New46EventsMessage/Associated TCMS Fault ID28 ==
  State : Inport
  Bus Creator1 : BusCreator  Inputs=2  OutDataTypeStr=Bus: BD_TCMSSystem_Out_Vehicle_Display_Message  NonVirtualBus=on
  Constant : Constant  Value=MessageID
  Data Type Conversion : DataTypeConversion
  Message : Outport  VectorParamsAs1DForOutWhenUnconnected=off
  wires:
  Data Type Conversion/1 -> Bus Creator1/2  "MessageStatus"
  Constant/1 -> Bus Creator1/1  "MessageID"
  State/1 -> Data Type Conversion/1
  Bus Creator1/1 -> Message/1

== system TCMSSystem/TCMSSystemPerVehicle/EnabledTCMSVehicle/OutputsPacking/TCMSDisplayOutputs/TCMSMessageEvents/New46EventsMessage/Associated TCMS Fault ID29 ==
  State : Inport
  Bus Creator1 : BusCreator  Inputs=2  OutDataTypeStr=Bus: BD_TCMSSystem_Out_Vehicle_Display_Message  NonVirtualBus=on
  Constant : Constant  Value=MessageID
  Data Type Conversion : DataTypeConversion
  Message : Outport  VectorParamsAs1DForOutWhenUnconnected=off
  wires:
  Bus Creator1/1 -> Message/1
  State/1 -> Data Type Conversion/1
  Constant/1 -> Bus Creator1/1  "MessageID"
  Data Type Conversion/1 -> Bus Creator1/2  "MessageStatus"

== system TCMSSystem/TCMSSystemPerVehicle/EnabledTCMSVehicle/OutputsPacking/TCMSDisplayOutputs/TCMSMessageEvents/New46EventsMessage/Associated TCMS Fault ID3 ==
  State : Inport
  Bus Creator1 : BusCreator  Inputs=2  OutDataTypeStr=Bus: BD_TCMSSystem_Out_Vehicle_Display_Message  NonVirtualBus=on
  Constant : Constant  Value=MessageID
  Data Type Conversion : DataTypeConversion
  Message : Outport  VectorParamsAs1DForOutWhenUnconnected=off
  wires:
  Bus Creator1/1 -> Message/1
  State/1 -> Data Type Conversion/1
  Constant/1 -> Bus Creator1/1  "MessageID"
  Data Type Conversion/1 -> Bus Creator1/2  "MessageStatus"

== system TCMSSystem/TCMSSystemPerVehicle/EnabledTCMSVehicle/OutputsPacking/TCMSDisplayOutputs/TCMSMessageEvents/New46EventsMessage/Associated TCMS Fault ID30 ==
  State : Inport
  Bus Creator1 : BusCreator  Inputs=2  OutDataTypeStr=Bus: BD_TCMSSystem_Out_Vehicle_Display_Message  NonVirtualBus=on
  Constant : Constant  Value=MessageID
  Data Type Conversion : DataTypeConversion
  Message : Outport  VectorParamsAs1DForOutWhenUnconnected=off
  wires:
  Data Type Conversion/1 -> Bus Creator1/2  "MessageStatus"
  Constant/1 -> Bus Creator1/1  "MessageID"
  State/1 -> Data Type Conversion/1
  Bus Creator1/1 -> Message/1

== system TCMSSystem/TCMSSystemPerVehicle/EnabledTCMSVehicle/OutputsPacking/TCMSDisplayOutputs/TCMSMessageEvents/New46EventsMessage/Associated TCMS Fault ID31 ==
  State : Inport
  Bus Creator1 : BusCreator  Inputs=2  OutDataTypeStr=Bus: BD_TCMSSystem_Out_Vehicle_Display_Message  NonVirtualBus=on
  Constant : Constant  Value=MessageID
  Data Type Conversion : DataTypeConversion
  Message : Outport  VectorParamsAs1DForOutWhenUnconnected=off
  wires:
  Bus Creator1/1 -> Message/1
  State/1 -> Data Type Conversion/1
  Constant/1 -> Bus Creator1/1  "MessageID"
  Data Type Conversion/1 -> Bus Creator1/2  "MessageStatus"

== system TCMSSystem/TCMSSystemPerVehicle/EnabledTCMSVehicle/OutputsPacking/TCMSDisplayOutputs/TCMSMessageEvents/New46EventsMessage/Associated TCMS Fault ID34 ==
  State : Inport
  Bus Creator1 : BusCreator  Inputs=2  OutDataTypeStr=Bus: BD_TCMSSystem_Out_Vehicle_Display_Message  NonVirtualBus=on
  Constant : Constant  Value=MessageID
  Data Type Conversion : DataTypeConversion
  Message : Outport  VectorParamsAs1DForOutWhenUnconnected=off
  wires:
  Bus Creator1/1 -> Message/1
  State/1 -> Data Type Conversion/1
  Constant/1 -> Bus Creator1/1  "MessageID"
  Data Type Conversion/1 -> Bus Creator1/2  "MessageStatus"

== system TCMSSystem/TCMSSystemPerVehicle/EnabledTCMSVehicle/OutputsPacking/TCMSDisplayOutputs/TCMSMessageEvents/New46EventsMessage/Associated TCMS Fault ID37 ==
  State : Inport
  Bus Creator1 : BusCreator  Inputs=2  OutDataTypeStr=Bus: BD_TCMSSystem_Out_Vehicle_Display_Message  NonVirtualBus=on
  Constant : Constant  Value=MessageID
  Data Type Conversion : DataTypeConversion
  Message : Outport  VectorParamsAs1DForOutWhenUnconnected=off
  wires:
  Bus Creator1/1 -> Message/1
  State/1 -> Data Type Conversion/1
  Constant/1 -> Bus Creator1/1  "MessageID"
  Data Type Conversion/1 -> Bus Creator1/2  "MessageStatus"

== system TCMSSystem/TCMSSystemPerVehicle/EnabledTCMSVehicle/OutputsPacking/TCMSDisplayOutputs/TCMSMessageEvents/New46EventsMessage/Associated TCMS Fault ID4 ==
  State : Inport
  Bus Creator1 : BusCreator  Inputs=2  OutDataTypeStr=Bus: BD_TCMSSystem_Out_Vehicle_Display_Message  NonVirtualBus=on
  Constant : Constant  Value=MessageID
  Data Type Conversion : DataTypeConversion
  Message : Outport  VectorParamsAs1DForOutWhenUnconnected=off
  wires:
  Data Type Conversion/1 -> Bus Creator1/2  "MessageStatus"
  Constant/1 -> Bus Creator1/1  "MessageID"
  State/1 -> Data Type Conversion/1
  Bus Creator1/1 -> Message/1

== system TCMSSystem/TCMSSystemPerVehicle/EnabledTCMSVehicle/OutputsPacking/TCMSDisplayOutputs/TCMSMessageEvents/New46EventsMessage/Associated TCMS Fault ID41 ==
  State : Inport
  Bus Creator1 : BusCreator  Inputs=2  OutDataTypeStr=Bus: BD_TCMSSystem_Out_Vehicle_Display_Message  NonVirtualBus=on
  Constant : Constant  Value=MessageID
  Data Type Conversion : DataTypeConversion
  Message : Outport  VectorParamsAs1DForOutWhenUnconnected=off
  wires:
  Bus Creator1/1 -> Message/1
  State/1 -> Data Type Conversion/1
  Constant/1 -> Bus Creator1/1  "MessageID"
  Data Type Conversion/1 -> Bus Creator1/2  "MessageStatus"
